simulink model "fifo8"  (Simulink 7.3)
settings: Solver=ode45  StartTime=0.0  StopTime=1000  RelTol=1e-3
libraries: simeventsgenerators1 x3, simeventssink1 x1, simeventsqueue1 x1, simeventsserver1 x1
settings Model: Creator=Roman  LastModifiedBy=Roman
settings SimEventsCC: propDiagAttribOutput=1  propDiagFcnCallOutput=1  propDiagStatOutput=0

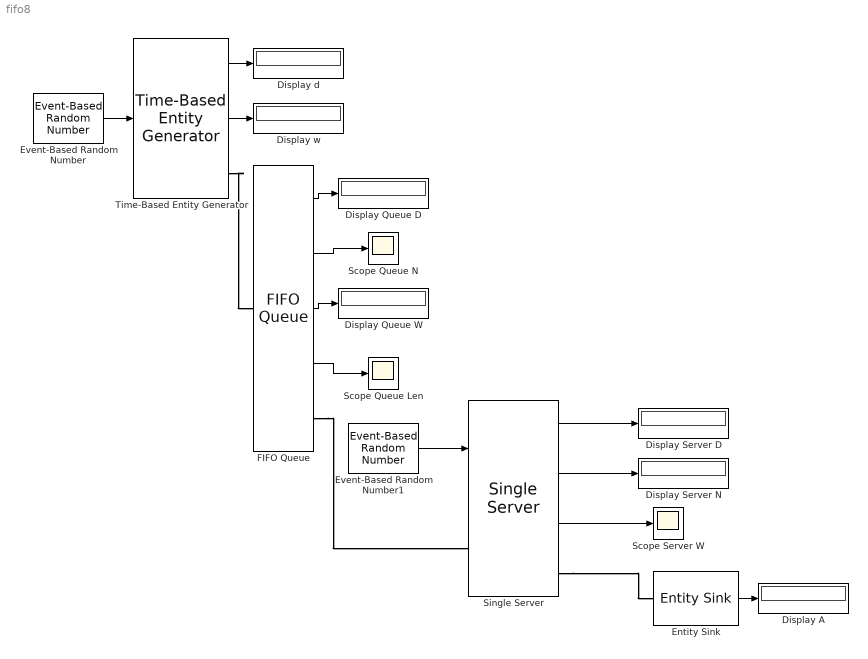
== system fifo8 ==
  Display A : Display
  Display Queue D : Display
  Display Queue W : Display
  Display Server D : Display
  Display Server N : Display
  Display d : Display
  Display w : Display
  Entity Sink : simeventssink1/Entity Sink  Priority=1  SystemSampleTime=-1  AvailableForArrivals=on  StatNumberArrived=On
  Event-Based Random Number : simeventsgenerators1/Signal Generators/Event-Based Random Number  SystemSampleTime=-1  distribution=Exponential  meanExp=2  minUnif=1  maxUnif=1  pOneBern=0.25  pSuccessBino=0.5  numTrialBino=1  meanNorm=0  stdNorm=1  minTri=1  maxTri=3  modeTri=2  thresholdLogn=0  scaleLogn=1  shapeLogn=1  pSuccessGeo=0.5  meanPoiss=1  thresholdLogl=0  scaleLogl=1  thresholdGam=0  scaleGam=1  shapeGam=1  minBeta=0  maxBeta=1  shape1Beta=1  shape2Beta=1  minUnid=0  maxUnid=1  numValueUnid=2  thresholdWbl=0  scaleWbl=1  shapeWbl=1  valueVecCont=[0 1]  cdfVecCont=[0 1]  valueVecDisc=[0 1]  probVecDisc=[0.5 0.5]  seed=12345  IsProcessed=on  isConnected=1
  Event-Based Random Number1 : simeventsgenerators1/Signal Generators/Event-Based Random Number  SystemSampleTime=-1  distribution=Gamma  meanExp=1  minUnif=0  maxUnif=6  pOneBern=0.25  pSuccessBino=0.5  numTrialBino=1  meanNorm=0  stdNorm=1  minTri=1  maxTri=3  modeTri=2  thresholdLogn=0  scaleLogn=1  shapeLogn=1  pSuccessGeo=0.5  meanPoiss=1  thresholdLogl=0  scaleLogl=1  thresholdGam=0  scaleGam=0.5  shapeGam=4  minBeta=0  maxBeta=1  shape1Beta=1  shape2Beta=1  minUnid=0  maxUnid=1  numValueUnid=2  thresholdWbl=0  scaleWbl=1  shapeWbl=1  valueVecCont=[0 1]  cdfVecCont=[0 1]  valueVecDisc=[0 1]  probVecDisc=[0.5 0.5]  seed=54321  IsProcessed=on  isConnected=1
  FIFO Queue : simeventsqueue1/FIFO Queue  Priority=1  SystemSampleTime=-1  Capacity=8  EnableTOPort=off  StatNumberDeparted=On  StatNumberInBlock=On  StatPendingEntity=Off  StatAverageWait=On  StatAverageQueueLength=On  StatNumberTimedout=Off
  Scope Queue Len : Scope
      settings: SaveName=LenQueue  DataFormat=Array
  Scope Queue N : Scope
      settings: SaveName=Nqueue  DataFormat=Array
  Scope Server W : Scope
      settings: SaveName=WServer  DataFormat=Array
  Single Server : simeventsserver1/Single Server  Priority=1  SystemSampleTime=-1  ServiceTimeFrom=Signal port t  ServiceTime=1  AttributeName=ServiceTime  PriorityServiceCompletion=500  PermitPreemption=off  SortingAttributeName=PriorityAttributeName  SortingDirection=Ascending  WriteToAttribute=off  ResidualAttributeName=ResidualServiceTime  CreateAttribute=on  EnableTOPort=off  StatNumberDeparted=On  StatNumberInBlock=On  StatNumberPreempted=Off  StatPendingEntity=Off  StatAverageWait=On  StatUtilization=Off  StatNumberTimedout=Off
  Time-Based Entity Generator : simeventsgenerators1/Entity Generators/Time-Based Entity Generator  Priority=1  DialogController=des_ddg_create  DialogControllerArgs=DataTag4  SystemSampleTime=-1  GenerateEntitiesUpon=Intergeneration time from port t  Distribution=Constant  Minimum=0  Maximum=1  Mean=1  InitialSeed=12345  Period=1  PriorityEntityGeneration=300  GenerateEntityAtSimulationStart=on  ResponseWhenBlocked=Pause generation  ResponseWhenUnblocked=Immediate restart  EntityType=Blank  StatNumberDeparted=On  StatPendingEntity=Off  StatAverageIntergenerationTime=On
  wires:
  Event-Based Random Number/1 -> Time-Based Entity Generator/1
  Time-Based Entity Generator/1 -> Display d/1
  Time-Based Entity Generator/2 -> Display w/1
  Single Server/3 -> Scope Server W/1
  Single Server/2 -> Display Server N/1
  Single Server/1 -> Display Server D/1
  Event-Based Random Number1/1 -> Single Server/1
  Entity Sink/1 -> Display A/1
  FIFO Queue/1 -> Display Queue D/1
  FIFO Queue/2 -> Scope Queue N/1
  FIFO Queue/3 -> Display Queue W/1
  FIFO Queue/4 -> Scope Queue Len/1
  connections:
  Time-Based Entity Generator/RConn1 -- FIFO Queue/LConn1
  Single Server/RConn1 -- Entity Sink/LConn1
  FIFO Queue/RConn1 -- Single Server/LConn1
